simulink model "dc_controller"  (R2022b)
settings: Solver=ode1  StartTime=0.0  StopTime=10.0  FixedStep=0.01  RelTol=1e-3
undefined symbols (not defined in the file or in its folder): DiscIntNeverNeededParam
libraries: simulink x1
settings Model: Creator=user  LastModifiedBy=user
settings OptimizationCC: DefaultParameterBehavior=Inlined  EnhancedBackFolding=on  PassReuseOutputArgsAs=Individual arguments  ZeroExternalMemoryAtStartup=off  ZeroInternalMemoryAtStartup=off  OptimizeBlockOrder=speed  DifferentSizesBufferReuse=on  OptimizationCustomize=off  EfficientTunableParamExpr=on
settings DebuggingCC: ParameterTunabilityLossMsg=error
settings SFSimCC: MATLABDynamicMemAlloc=off
settings RTWCC: Description=Embedded Coder  SystemTargetFile=ert.tlc  TemplateMakefile=ert_default_tmf
settings CodeAppCC: ForceParamTrailComments=on  IgnoreCustomStorageClasses=off  OperatorAnnotations=on  SimulinkDataObjDesc=on  SFDataObjDesc=on  InsertBlockDesc=on
settings ERTTargetCC: TargetLangStandard=C99 (ISO)  GenerateSampleERTMain=on  InlinedParameterPlacement=NonHierarchical  ERTCustomFileTemplate=example_file_process.tlc

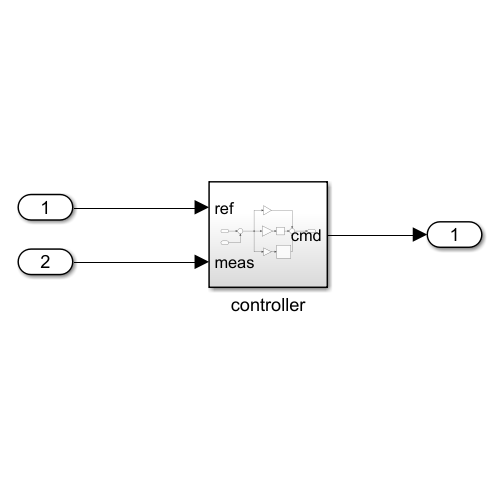
[thumbnail: Simulink's stored preview of the top-level diagram]
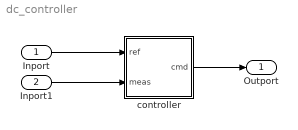
== system dc_controller ==
  Inport : Inport
  Inport1 : Inport  Port=2
  controller : Subsystem
  Outport : Outport
  wires:
  Inport/1 -> controller/1(ref)
  Inport1/1 -> controller/2(meas)
  controller/1(cmd) -> Outport/1

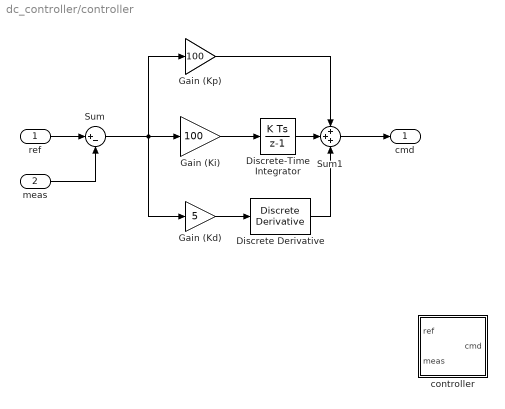
== system dc_controller/controller ==
  ref : Inport
  meas : Inport  Port=2
  Discrete Derivative : simulink/Discrete/Discrete Derivative  gainval=1.0  ICPrevScaledInput=0.0  OutMin=[]  OutMax=[]  OutDataType=fixdt(1, 16)  OutScaling=2^-10  DoSatur=off
  Discrete-Time Integrator : DiscreteIntegrator  SampleTime=-1  ICPrevOutput=DiscIntNeverNeededParam  ICPrevScaledInput=DiscIntNeverNeededParam
  Gain (Kd) : Gain  Gain=5
  Gain (Ki) : Gain  Gain=100
  Gain (Kp) : Gain  Gain=100
  Sum : Sum  Inputs=|+-
  Sum1 : Sum  Inputs=+++
  controller : Subsystem
  cmd : Outport
  wires:
  Discrete-Time Integrator/1 -> Sum1/2
  Discrete Derivative/1 -> Sum1/3
  Sum/1 -> Gain (Kp)/1, Gain (Ki)/1, Gain (Kd)/1
  ref/1 -> Sum/1
  meas/1 -> Sum/2
  Gain (Ki)/1 -> Discrete-Time Integrator/1
  Gain (Kd)/1 -> Discrete Derivative/1
  Sum1/1 -> cmd/1
  Gain (Kp)/1 -> Sum1/1

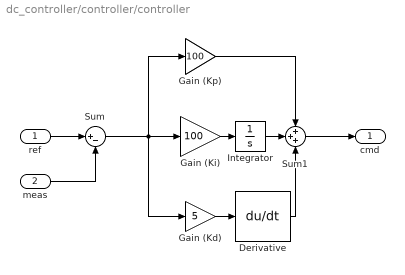
== system dc_controller/controller/controller ==
  ref : Inport
  meas : Inport  Port=2
  Derivative : Derivative
  Gain (Kd) : Gain  Gain=5
  Gain (Ki) : Gain  Gain=100
  Gain (Kp) : Gain  Gain=100
  Integrator : Integrator
  Sum : Sum  Inputs=|+-
  Sum1 : Sum  Inputs=+++
  cmd : Outport
  wires:
  Integrator/1 -> Sum1/2
  Derivative/1 -> Sum1/3
  Sum/1 -> Gain (Kp)/1, Gain (Ki)/1, Gain (Kd)/1
  ref/1 -> Sum/1
  meas/1 -> Sum/2
  Gain (Ki)/1 -> Integrator/1
  Gain (Kd)/1 -> Derivative/1
  Sum1/1 -> cmd/1
  Gain (Kp)/1 -> Sum1/1
